simulink library "RobotStateLibrary"  (R2021b)
settings: Solver=VariableStepAuto  StartTime=0.0  StopTime=10.0  RelTol=1e-3
undefined symbols (not defined in the file or in its folder): Aeq_add, baseFrameName1, basePosePortName, beq_add, config, Config, ConfigRobot1, configSafety, contactFrame1Name, contactFrame2Name, frame1, frame2, frame3, frame4, frameName1, frameName2, gainStruct, RegStruct, regularization, sampleTime, tollerance, useConstraint, weight
libraries: WBToolboxLibrary x36, $bdroot x34, spsFirstOrderFilterLib x1, simulink x1
(part 2 of 2)

== system RobotStateLibrary/emergency stop: joint limits/STOP IF THERE ARE SPIKES IN THE ENCODERS ==
  jointPos : Inport
  Enable : EnablePort
  Assertion : Assertion
  MATLAB Function : MATLAB Function  TreatAsAtomicUnit=on
  Unit Delay : UnitDelay  InitialCondition=1  SampleTime=Config.tStep  HasFrameUpgradeWarning=on
  index1 : Constant  Value=Safety.maxJointsPositionDelta  VectorParams1D=off
  check_spikes_joint_pos : Outport
  wires:
  jointPos/1 -> MATLAB Function/1(u)
  MATLAB Function/1(noSpikes) -> Unit Delay/1
  index1/1 -> MATLAB Function/2(delta_u_max)
  MATLAB Function/2(res_check_spikes) -> check_spikes_joint_pos/1
  Unit Delay/1 -> Assertion/1

== matlab function RobotStateLibrary/Compute Base Transform from two links/Rotation Average ==
  data: w_H_1 input; w_H output; w_H_2 input
function w_H = rotationAverageFCN(w_H_1, w_H_2)

w_H = rsl.rotationAverage(w_H_1, w_H_2);

end

== matlab function RobotStateLibrary/Compute State Velocity/Compute Base Velocity ==
  data: J_contact_1 input; J_contact_2 input; nu_b output; jointVel input; regularization parameter
function nu_b = computeBaseVelocityFCN(J_contact_1, J_contact_2, jointVel, regularization)

    nu_b = rsl.computeBaseVelocityFromContacts(J_contact_1, J_contact_2, jointVel, regularization);

end

== matlab function RobotStateLibrary/Force Ergonomy Optimization/Pseudoinverse ==
  data: Aeq input; yMinNorm output; beq input; null output; InvTol parameter
function [yMinNorm, null] = pseudoinverseFCN(Aeq, beq, InvTol)

[yMinNorm, null] = rsl.pseudoinverse(Aeq, beq, InvTol);

end

== matlab function RobotStateLibrary/Force Ergonomy Optimization/Prepare QP optimization ==
  data: yMinNorm input; H output; null input; tau_model input; tau_sigma input; Adeq input; bdeq input; yDes input; g output; A output; ubA output; regularizationHessian parameter; minimizationWeight parameter; regularizationYDes parameter
function [H, g, A, ubA] = prepareQPOptimizationFCN(yMinNorm, null, tau_model, tau_sigma, Adeq, bdeq, yDes, regularizationHessian, minimizationWeight, regularizationYDes)

[H, g, A, ubA] = rsl.prepareQPOptimization(yMinNorm, null, tau_model, tau_sigma, Adeq, bdeq, yDes, regularizationHessian, regularizationYDes, minimizationWeight);

end

== matlab function RobotStateLibrary/State-Machine Reference Generator with Parametrization/State-Machine ==
  data: jointPos input; nu input; jointPos_des output; jointVel_des output; posCoM input; time input; J input; linkPose input; linkPoseDes input; linkVelocityDes input; posCoM_des output; configStateMachine parameter; useForwardKinematicsForCoM output; phi output; currentState output
function [jointPos_des, jointVel_des, posCoM_des, useForwardKinematicsForCoM, phi, currentState] = stateMachineTimeParametrizedFCN(jointPos, nu, posCoM, time, J, linkPose, linkPoseDes, linkVelocityDes, configStateMachine)

[jointPos_des, jointVel_des, posCoM_des, useForwardKinematicsForCoM, phi, currentState] = rsl.stateMachineTimeParametrized(jointPos, nu, posCoM, time, J, linkPose, linkPoseDes, linkVelocityDes, configStateMachine);

end

== matlab function RobotStateLibrary/emergency stop: joint limits/STOP IF REQUESTED JOINT TORQUES REACH THE LIMITS/MATLAB Function ==
  data: umin input; umax input; u input; inRange output; tol input; res_check_range output
function [inRange, res_check_range] = checkInputRangeFCN(umin, umax, u, tol)

     [inRange, res_check_range] = wbc.checkInputRange(umin, umax, u, tol);
end

== matlab function RobotStateLibrary/Unscent Kalman Filter/MATLAB Function ==
  data: x_meas input; x output; x_dot_meas input; x_dot output; x_ddot output; P output; dt input
function [x, x_dot, x_ddot, P] = UKF_FCN(x_meas, x_dot_meas, dt)

persistent ukf
persistent Xs
persistent Px
persistent f_trans
persistent f_meas

if isempty(ukf)
    Xs = [0.0, 0.0, 0.0];
    Px = [1.0, 1.0, 1.0];
    f_trans = @(x, u) transition_fun(x, u, dt); % u=0
    f_meas = @(x) measurement_fun(x);

    ukf = iRonCubLib.UKF("f_meas", f_meas, ...
              "f_trans", f_trans, ...
              "initial_covariance", eye(3) * 1e0, ...
              "measurement_noise", diag([0.05, 0.1]), ...
              "process_noise", diag([1e-3, 1e-5, 1e-2]));
end


[Xs, P] = ukf.step(Xs, 0, [x_meas; x_dot_meas]);

x = Xs(1);
x_dot = Xs(2);
x_ddot = Xs(3);

function x = transition_fun(x, u, dt)
    % simple kinematic model
    A = [1, dt, dt^2/2;...
         0, 1,  dt; ...
         0, 0,  1];

    x = A * x;
end

function y = measurement_fun(x)
    y = [x(1); x(2)];
end


end

== matlab function RobotStateLibrary/emergency stop: joint limits/STOP IF THERE ARE SPIKES IN THE ENCODERS/MATLAB Function ==
  data: u input; delta_u_max input; noSpikes output; res_check_spikes output
function [noSpikes, res_check_spikes] = checkInputSpikesFCN(u, delta_u_max)

     [noSpikes, res_check_spikes] = wbc.checkInputSpikes(u, delta_u_max);
end

== matlab function RobotStateLibrary/emergency stop: joint limits/STOP IF JOINTS HIT THE LIMITS/MATLAB Function ==
  data: umin input; umax input; u input; inRange output; tol input; res_check_range output
function [inRange, res_check_range] = checkInputRangeFCN(umin, umax, u, tol)

     [inRange, res_check_range] = wbc.checkInputRange(umin, umax, u, tol);
end

== matlab function RobotStateLibrary/Postural Task Controller/Postural Task Controller ==
  data: jointPos input; nu input; J input; tau_0_model output; M input; h input; jointPos_des input; jointVel_des input; tau_0_sigma output; GainPostural parameter
function [tau_0_model, tau_0_sigma] =  posturalTaskControllerFCN(jointPos, nu, J, M, h, jointPos_des, jointVel_des, GainPostural)

[tau_0_model, tau_0_sigma] = rsl.posturalTaskController(jointPos, nu, J, M, h, jointPos_des, jointVel_des, GainPostural);

end

== matlab function RobotStateLibrary/Pose Yarp Publisher/Transform Matrix to quaternion and position ==
  data: w_H input; q output
function q = transformMatrixToPositionQuaternion_FCN(w_H)

q = wbc.fromTransfMatrixToPosQuat(w_H);

== matlab function RobotStateLibrary/Momentum Controller/Momentum Controller Wrench ==
  data: L input; pos_CoM input; desired_pos_vel_acc_CoM input; w_H_meas input; w_R_des input; w_H_contacts input; mass input; wrench_Aeq output; wrench_beq output; wrench_Adeq output; wrench_bdeq output; constraintsMatrixA input; constraintsVectorb input; linksUseConstraintMatrix parameter; GainMomentum parameter
function [wrench_Aeq, wrench_beq, wrench_Adeq, wrench_bdeq] =  momentumControllerWrenchFCN(L, pos_CoM, desired_pos_vel_acc_CoM, w_H_meas, w_R_des, w_H_contacts, mass, constraintsMatrixA, constraintsVectorb, linksUseConstraintMatrix, GainMomentum)

[wrench_Aeq, wrench_beq, wrench_Adeq, wrench_bdeq] = rsl.momentumControllerWrench(L, pos_CoM, desired_pos_vel_acc_CoM, w_H_meas, w_R_des, w_H_contacts, mass, constraintsMatrixA, constraintsVectorb, linksUseConstraintMatrix, GainMomentum);

end

== matlab function RobotStateLibrary/Inverse Dynamics/Inverse Dynamics ==
  data: tau_model output; tau_0_model input; tau_0_sigma input; J input; JDot_nu input; M input; h input; B input; tau_sigma output; Reg parameter; fixedLinkVelcityComponents parameter; Lambda output
function [tau_model, tau_sigma, Lambda] = inverseDynamicsFCN(tau_0_model, tau_0_sigma, J, JDot_nu, M, h, B, Reg, fixedLinkVelcityComponents)

[tau_model, tau_sigma, Lambda] = rsl.inverseDynamics(tau_0_model, tau_0_sigma, J, JDot_nu, M, h, B, fixedLinkVelcityComponents, Reg);

end

== matlab function RobotStateLibrary/State-Machine Reference Generator/State-Machine ==
  data: jointPos input; jointPos_des output; posCoM input; time input; posCoM_des output; smoothingTime output; configStateMachine parameter; useSmoothing output; useForwardKinematicsForCoM output; currentState output
function [jointPos_des, posCoM_des, smoothingTime, useSmoothing, useForwardKinematicsForCoM, currentState] = stateMachineFCN(jointPos, posCoM, time, configStateMachine)

[jointPos_des, posCoM_des, smoothingTime, useSmoothing, useForwardKinematicsForCoM, currentState] = rsl.stateMachine(jointPos, posCoM, time, configStateMachine);

end
